simulink model "NewBlockFlow"  (R2021a)
settings: Solver=VariableStepAuto  StartTime=0.0  StopTime=10.0  RelTol=1e-3
values from neighbouring files (symbols this model uses):
  a = 0    [gainMaxDef.m]    (also in plot2.m = 2; simulink_test.m = 5)
  alpha = 1.195    [gainMaxDef.m]    (also in plot2.m = 1.9; simulink_test.m = 1.192)
  betac = 2    [plot2.m]    (also in simulink_test.m = 10)
  delay = 0.5    [plot2.m]    (also in simulink_test.m = 0.015)
  delay_a = 0.150    (= 0.15)    [plot2.m]    (also in simulink_test.m = 0.01)
  gnet = 40    [plot2.m]    (also in simulink_test.m = gnetset(k))
  omega = omegalist(l)    [gainMaxDef.m]    (also in plot2.m = 300; simulink_test.m = 0.8)
  omegader = 80    [simulink_test.m]
libraries: cstblocks x24, simulink x2
(part 1 of 2)
settings Model: Creator=shiva  LastModifiedBy=shiva

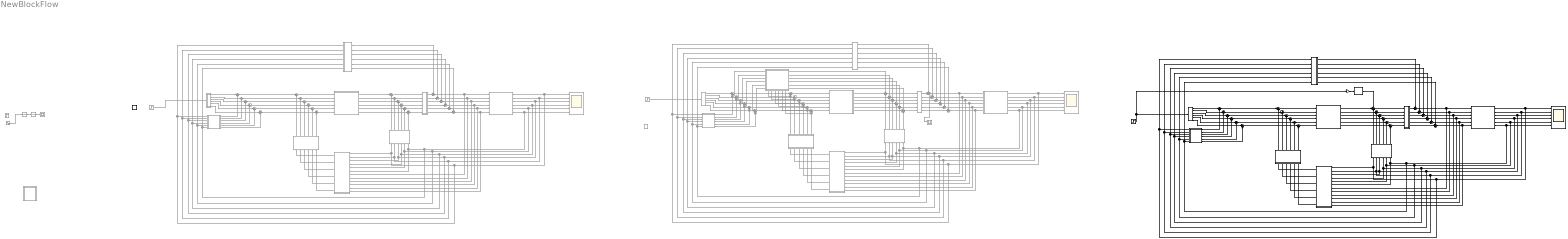
== system NewBlockFlow ==
  note: FLOW V3
  note: FLOW V2
  note: FLOW V1
  note: CONTROL BLOCK
  note: FEEDBACK
  note: INPUT AREA
  note: FEEDBACK
  note: CONTROL BLOCK
  note: INPUT AREA
  note: FEEDBACK
  note: CONTROL BLOCK
  note: INPUT AREA
  Adjency : Subsystem  Commented=on
  Adjency1 : Subsystem  Commented=on
  Adjency2 : Subsystem
  B : Subsystem  Commented=on
  B1 : Subsystem  Commented=on
  B2 : Subsystem
  C(s) : Subsystem  Commented=on
  C(s)1 : Subsystem  Commented=on
  C(s)2 : Subsystem
  CDOB_Subsys1 : Subsystem  Commented=on
  CDOB_Subsys2 : Subsystem
  CDOB_Subsys4 : Subsystem  Commented=on
  DSRdelayV2 : Subsystem
  Degree : Subsystem  Commented=on
  Degree1 : Subsystem  Commented=on
  Degree2 : Subsystem
  DerivativeEstimater : Subsystem  Commented=on
  DerivativeEstimater1 : Subsystem  Commented=on
  DerivativeEstimater2 : Subsystem
  G(s)e^(-tau*s) : Subsystem  Commented=on
  G(s)e^(-tau*s)1 : Subsystem  Commented=on
  G(s)e^(-tau*s)2 : Subsystem
  Gain : Gain  Gain=betac
  Identity : Subsystem  Commented=on
  PseudoDerivative : Subsystem  Commented=on
  Ramp : simulink/Sources/Ramp  slope=1  start=0  InitialOutput=0
  Ramp1 : simulink/Sources/Ramp  Commented=on  slope=1  start=0  InitialOutput=0
  Scope : Scope  Commented=on
  Scope1 : Scope  Commented=on  NumInputPorts=6
  Scope2 : Scope  Commented=on  NumInputPorts=2
  Scope3 : Scope  NumInputPorts=6
  Scope5 : Scope  Commented=on  NumInputPorts=6
  Sine Wave : Sin  Commented=on  SampleTime=0
  StateDerivative1 : Subsystem
  StateDerivative3 : Subsystem  Commented=on
  Step : Step  Commented=on  Time=0  SampleTime=0
  Step1 : Step  Commented=on  SampleTime=0
  Step2 : Step  Commented=on  Time=0  SampleTime=0
  Step3 : Step  Time=0  SampleTime=0
  Sum{,1..5,12..17,28..33} (18 alike) : Sum  Commented=on  Inputs=|++
  Sum{6..11,26..27,44..47} (12 alike) : Sum  Commented=on  Inputs=++|
  Sum{18..23,34..35,37..40} (12 alike) : Sum  Commented=on  Inputs=|-+
  Sum{24..25,36,41..43} (6 alike) : Sum  Commented=on  Inputs=-++
  Sum48 : Sum  Inputs=-++
  Sum{49,52..57,60,65..67} (11 alike) : Sum  Inputs=|++
  Sum{50..51,68..71} (6 alike) : Sum  Inputs=++|
  Sum{58..59,61..64} (6 alike) : Sum  Inputs=|-+
  beta*(DXc-Ax)*F(s) : Subsystem  Commented=on
      settings: PortSchema="{\"entries\":[{\"content\":{\"sides\":[{\"content\":{\"connectorIds\":[\"In1\",\"In2\",\"In3\",\"In4\",\"In5\",\"In6\"]},\"type\":\"ConnectorPlacement.EquallySpacedRectSide\",\"uuid\":\"7b965991-8f4b-4d23-8dac-1fc1cf204da0\"},{\"content\":{\"connectorIds\":[\"Out1\",\"Out2\",\"Out3\",\"Out4\",\"Out5\",\"Out6\"],\"side\":\"RIGHT\"},\"type\":\"ConnectorPlacement.EquallySpacedRectSide\",\"uuid\":\"f5ccf5a4-70bb-4fce-9767-13471ee96b32\"},{\"content\":{\"connectorIds\":[],\"side\":\"TOP\"},\"type\":\"ConnectorPlacement.EquallySpacedRectSide\",\"uuid\":\"af7cab47-c5e2-4c4a-b9c2-1fd2a05ea20b\"},{\"content\":{\"connectorIds\":[\"In7\",\"In8\",\"In9\",\"In10\",\"In11\",\"In12\"],\"side\":\"BOTTOM\"},\"type\":\"ConnectorPlacement.EquallySpacedRectSide\",\"uuid\":\"30ff81f8-6ce8-42b1-8056-7bce911790b7\"}]},\"type\":\"ConnectorPlacement.EquallySpacedConnector\",\"uuid\":\"9d803241-f085-403f-8915-bf1fb56b5898\"}],\"packageUris\":[\"http://schema.mathworks.com/mf0/Connector/R2020b\"],\"version\":\"1.0\"}"
  gain 1/a : Subsystem  Commented=on
  gain 1/a1 : Subsystem  Commented=on
  gain 1/a2 : Subsystem
  pseudoDer : TransferFcn  Commented=on  Numerator=[omegader 0]  Denominator=[1 omegader]
  pseudoDer1 : TransferFcn  Commented=on  Numerator=[omegader 0]  Denominator=[1 omegader]
  wires:
  G(s)e^(-tau*s)/1(pos) -> CDOB_Subsys4/1(XRes), DerivativeEstimater/1(pos), PseudoDerivative/1(Input), Adjency/1(Input), Scope5/1
  G(s)e^(-tau*s)/2(pos1) -> Scope5/2, PseudoDerivative/2(Input1), Adjency/2(Input1), CDOB_Subsys4/2(XRes1), DerivativeEstimater/2(pos1)
  G(s)e^(-tau*s)/3(pos2) -> Scope5/3, PseudoDerivative/3(Input2), Adjency/3(Input2), CDOB_Subsys4/3(XRes2), DerivativeEstimater/3(pos2)
  G(s)e^(-tau*s)/4(pos3) -> Scope5/4, PseudoDerivative/4(Input3), Adjency/4(Input3), CDOB_Subsys4/4(XRes3), DerivativeEstimater/4(pos3)
  G(s)e^(-tau*s)/5(pos4) -> Scope5/5, Adjency/5(Input4), PseudoDerivative/5(Input4), CDOB_Subsys4/5(XRes4), DerivativeEstimater/5(pos4)
  G(s)e^(-tau*s)/6(pos5) -> Scope5/6, CDOB_Subsys4/6(XRes5), DerivativeEstimater/6(pos5), PseudoDerivative/6(Input5), Adjency/6(Input5)
  DerivativeEstimater/1(est) -> Sum/2
  C(s)/1(Out1) -> Sum/1
  Sum6/1 -> CDOB_Subsys4/7(Acc.), G(s)e^(-tau*s)/1(In1)
  Sum7/1 -> CDOB_Subsys4/8(Acc.1), G(s)e^(-tau*s)/2(In2)
  C(s)/2(Out2) -> Sum1/1
  DerivativeEstimater/3(est2) -> Sum2/2
  C(s)/3(Out3) -> Sum2/1
  Sum8/1 -> CDOB_Subsys4/9(Acc.2), G(s)e^(-tau*s)/3(In3)
  DerivativeEstimater/4(est3) -> Sum3/2
  Sum9/1 -> CDOB_Subsys4/10(Acc.3), G(s)e^(-tau*s)/4(In4)
  C(s)/4(Out4) -> Sum3/1
  DerivativeEstimater/5(est4) -> Sum4/2
  C(s)/5(Out5) -> Sum4/1
  Sum10/1 -> CDOB_Subsys4/11(Acc.4), G(s)e^(-tau*s)/5(In5)
  DerivativeEstimater/6(est5) -> Sum5/2
  C(s)/6(Out6) -> Sum5/1
  Sum11/1 -> CDOB_Subsys4/12(Acc.5), G(s)e^(-tau*s)/6(In6)
  DerivativeEstimater/2(est1) -> Sum1/2
  gain 1/a/1(Out1) -> Sum6/2
  gain 1/a/2(Out2) -> Sum7/2
  gain 1/a/3(Out3) -> Sum8/2
  gain 1/a/4(Out4) -> Sum9/2
  gain 1/a/5(Out5) -> Sum10/2
  gain 1/a/6(Out6) -> Sum11/2
  Sum/1 -> gain 1/a/1(In1)
  Sum1/1 -> gain 1/a/2(In2)
  Sum2/1 -> gain 1/a/3(In3)
  Sum3/1 -> gain 1/a/4(In4)
  Sum4/1 -> gain 1/a/5(In5)
  Sum5/1 -> gain 1/a/6(In6)
  Step/1 -> B/1(Input)
  B/1(Output) -> Sum12/1
  Adjency/1(Output) -> Sum12/2
  B/2(Output1) -> Sum13/1
  B/3(Output2) -> Sum14/1
  B/4(Output3) -> Sum15/1
  B/5(Output4) -> Sum16/1
  B/6(Output5) -> Sum17/1
  Adjency/2(Output1) -> Sum13/2
  Adjency/3(Output2) -> Sum14/2
  Adjency/4(Output3) -> Sum15/2
  Adjency/5(Output4) -> Sum16/2
  Adjency/6(Output5) -> Sum17/2
  Sum12/1 -> Sum18/1
  Sum18/1 -> C(s)/1(R-F)
  Sum19/1 -> C(s)/2(R-F1)
  Sum20/1 -> C(s)/3(R-F2)
  Sum21/1 -> C(s)/4(R-F3)
  Sum22/1 -> C(s)/5(R-F4)
  Sum23/1 -> C(s)/6(R-F5)
  Sum13/1 -> Sum19/1
  Sum14/1 -> Sum20/1
  Sum15/1 -> Sum21/1
  Sum16/1 -> Sum22/1
  Sum17/1 -> Sum23/1
  CDOB_Subsys4/1(FeedBack) -> Degree/1(Input)
  CDOB_Subsys4/2(FeedBack1) -> Degree/2(Input1)
  CDOB_Subsys4/3(FeedBack2) -> Degree/3(Input2)
  CDOB_Subsys4/4(FeedBack3) -> Degree/4(Input3)
  CDOB_Subsys4/5(FeedBack4) -> Degree/5(Input4)
  CDOB_Subsys4/6(FeedBack5) -> Degree/6(Input5)
  Degree/1(Output) -> Sum18/2
  Degree/6(Output5) -> Sum23/2
  Degree/5(Output4) -> Sum22/2
  Degree/4(Output3) -> Sum21/2
  Degree/3(Output2) -> Sum20/2
  Degree/2(Output1) -> Sum19/2
  PseudoDerivative/1(Output) -> Sum6/1
  PseudoDerivative/2(Output1) -> Sum7/1
  PseudoDerivative/3(Output2) -> Sum8/1
  PseudoDerivative/4(Output3) -> Sum9/1
  PseudoDerivative/5(Output4) -> Sum10/1
  PseudoDerivative/6(Output5) -> Sum11/1
  pseudoDer/1 -> pseudoDer1/1
  pseudoDer1/1 -> Scope/1
  Sine Wave/1 -> pseudoDer/1
  Step2/1 -> B1/1(Input)
  StateDerivative3/1(Out1) -> Sum44/1
  StateDerivative3/6(Out6) -> Sum27/1
  StateDerivative3/3(Out3) -> Sum46/1
  StateDerivative3/2(Out2) -> Sum45/1
  Degree1/2(Output1) -> beta*(DXc-Ax)*F(s)/8(Input7), Sum35/2
  CDOB_Subsys1/6(FeedBack5) -> Degree1/6(Input5)
  Adjency1/5(Output4) -> beta*(DXc-Ax)*F(s)/5(Input4), Sum32/2
  B1/4(Output3) -> Sum31/1
  StateDerivative3/5(Out5) -> Sum26/1
  B1/1(Output) -> Sum28/1
  Sum34/1 -> C(s)1/1(R-F)
  Sum32/1 -> Sum39/1
  Degree1/5(Output4) -> beta*(DXc-Ax)*F(s)/11(Input10), Sum39/2
  Adjency1/3(Output2) -> beta*(DXc-Ax)*F(s)/3(Input2), Sum30/2
  B1/2(Output1) -> Sum29/1
  Sum38/1 -> C(s)1/4(R-F3)
  B1/6(Output5) -> Sum33/1
  Sum29/1 -> Sum35/1
  Adjency1/4(Output3) -> beta*(DXc-Ax)*F(s)/4(Input3), Sum31/2
  Sum30/1 -> Sum37/1
  Sum33/1 -> Sum40/1
  B1/5(Output4) -> Sum32/1
  Adjency1/2(Output1) -> beta*(DXc-Ax)*F(s)/2(Input1), Sum29/2
  Sum40/1 -> C(s)1/6(R-F5)
  G(s)e^(-tau*s)1/5(pos4) -> Scope1/5, Adjency1/5(Input4), StateDerivative3/5(Input4), CDOB_Subsys1/5(XRes4), DerivativeEstimater1/5(pos4)
  Sum27/1 -> CDOB_Subsys1/12(Acc.5), G(s)e^(-tau*s)1/6(In6)
  G(s)e^(-tau*s)1/3(pos2) -> Scope1/3, StateDerivative3/3(Input2), Adjency1/3(Input2), CDOB_Subsys1/3(XRes2), DerivativeEstimater1/3(pos2)
  Degree1/6(Output5) -> beta*(DXc-Ax)*F(s)/12(Input11), Sum40/2
  G(s)e^(-tau*s)1/4(pos3) -> Scope1/4, StateDerivative3/4(Input3), Adjency1/4(Input3), CDOB_Subsys1/4(XRes3), DerivativeEstimater1/4(pos3)
  G(s)e^(-tau*s)1/1(pos) -> CDOB_Subsys1/1(XRes), DerivativeEstimater1/1(pos), StateDerivative3/1(Input), Adjency1/1(Input), Scope1/1
  Sum47/1 -> CDOB_Subsys1/10(Acc.3), G(s)e^(-tau*s)1/4(In4)
  Degree1/4(Output3) -> beta*(DXc-Ax)*F(s)/10(Input9), Sum38/2
  CDOB_Subsys1/2(FeedBack1) -> Degree1/2(Input1)
  gain 1/a1/3(Out3) -> Sum46/2
  G(s)e^(-tau*s)1/6(pos5) -> Scope1/6, CDOB_Subsys1/6(XRes5), DerivativeEstimater1/6(pos5), StateDerivative3/6(Input5), Adjency1/6(Input5)
  gain 1/a1/6(Out6) -> Sum27/2
  Sum31/1 -> Sum38/1
  gain 1/a1/2(Out2) -> Sum45/2
  Sum28/1 -> Sum34/1
  Sum26/1 -> CDOB_Subsys1/11(Acc.4), G(s)e^(-tau*s)1/5(In5)
  Sum45/1 -> CDOB_Subsys1/8(Acc.1), G(s)e^(-tau*s)1/2(In2)
  Degree1/1(Output) -> beta*(DXc-Ax)*F(s)/7(Input6), Sum34/2
  Sum24/1 -> gain 1/a1/1(In1)
  Sum46/1 -> CDOB_Subsys1/9(Acc.2), G(s)e^(-tau*s)1/3(In3)
  StateDerivative3/4(Out4) -> Sum47/1
  CDOB_Subsys1/4(FeedBack3) -> Degree1/4(Input3)
  Sum39/1 -> C(s)1/5(R-F4)
  B1/3(Output2) -> Sum30/1
  Sum37/1 -> C(s)1/3(R-F2)
  G(s)e^(-tau*s)1/2(pos1) -> Scope1/2, StateDerivative3/2(Input1), Adjency1/2(Input1), CDOB_Subsys1/2(XRes1), DerivativeEstimater1/2(pos1)
  gain 1/a1/1(Out1) -> Sum44/2
  CDOB_Subsys1/3(FeedBack2) -> Degree1/3(Input2)
  Degree1/3(Output2) -> beta*(DXc-Ax)*F(s)/9(Input8), Sum37/2
  gain 1/a1/4(Out4) -> Sum47/2
  Sum44/1 -> Scope2/1, CDOB_Subsys1/7(Acc.), G(s)e^(-tau*s)1/1(In1)
  Sum35/1 -> C(s)1/2(R-F1)
  CDOB_Subsys1/1(FeedBack) -> Degree1/1(Input)
  gain 1/a1/5(Out5) -> Sum26/2
  CDOB_Subsys1/5(FeedBack4) -> Degree1/5(Input4)
  Adjency1/1(Output) -> beta*(DXc-Ax)*F(s)/1(Input), Sum28/2
  Adjency1/6(Output5) -> beta*(DXc-Ax)*F(s)/6(Input5), Sum33/2
  Sum43/1 -> gain 1/a1/6(In6)
  Sum25/1 -> gain 1/a1/2(In2)
  Sum36/1 -> gain 1/a1/3(In3)
  Sum41/1 -> gain 1/a1/4(In4)
  Sum42/1 -> gain 1/a1/5(In5)
  beta*(DXc-Ax)*F(s)/1(Output) -> Sum24/1
  DerivativeEstimater1/1(est) -> Sum24/3
  DerivativeEstimater1/6(est5) -> Sum43/3
  C(s)1/6(Out6) -> Sum43/2
  DerivativeEstimater1/5(est4) -> Sum42/3
  C(s)1/5(Out5) -> Sum42/2
  C(s)1/4(Out4) -> Sum41/2
  DerivativeEstimater1/4(est3) -> Sum41/3
  DerivativeEstimater1/3(est2) -> Sum36/3
  C(s)1/3(Out3) -> Sum36/2
  DerivativeEstimater1/2(est1) -> Sum25/3
  C(s)1/2(Out2) -> Sum25/2
  C(s)1/1(Out1) -> Sum24/2
  beta*(DXc-Ax)*F(s)/2(Output1) -> Sum25/1
  beta*(DXc-Ax)*F(s)/3(Output2) -> Sum36/1
  beta*(DXc-Ax)*F(s)/4(Output3) -> Sum41/1
  beta*(DXc-Ax)*F(s)/5(Output4) -> Sum42/1
  beta*(DXc-Ax)*F(s)/6(Output5) -> Sum43/1
  Step3/1 -> Gain/1, B2/1(Input)
  StateDerivative1/1(Out1) -> Sum68/1
  StateDerivative1/6(Out6) -> Sum51/1
  StateDerivative1/3(Out3) -> Sum70/1
  StateDerivative1/2(Out2) -> Sum69/1
  Degree2/2(Output1) -> Sum59/2
  CDOB_Subsys2/6(FeedBack5) -> Degree2/6(Input5)
  Adjency2/5(Output4) -> Sum56/2
  B2/4(Output3) -> Sum55/1
  StateDerivative1/5(Out5) -> Sum50/1
  B2/1(Output) -> Sum52/1
  Sum58/1 -> C(s)2/1(R-F)
  Sum56/1 -> Sum63/1
  Degree2/5(Output4) -> Sum63/2
  Adjency2/3(Output2) -> Sum54/2
  B2/2(Output1) -> Sum53/1
  Sum62/1 -> C(s)2/4(R-F3)
  B2/6(Output5) -> Sum57/1
  Sum53/1 -> Sum59/1
  Adjency2/4(Output3) -> Sum55/2
  Sum54/1 -> Sum61/1
  Sum57/1 -> Sum64/1
  B2/5(Output4) -> Sum56/1
  Adjency2/2(Output1) -> Sum53/2
  Sum64/1 -> C(s)2/6(R-F5)
  Sum66/1 -> gain 1/a2/5(In5)
  G(s)e^(-tau*s)2/5(pos4) -> Scope3/5, Adjency2/5(Input4), StateDerivative1/5(Input4), CDOB_Subsys2/5(XRes4), DerivativeEstimater2/5(pos4)
  DerivativeEstimater2/6(est5) -> Sum67/2
  C(s)2/5(Out5) -> Sum66/1
  Sum51/1 -> CDOB_Subsys2/12(Acc.5), G(s)e^(-tau*s)2/6(In6)
  G(s)e^(-tau*s)2/3(pos2) -> Scope3/3, StateDerivative1/3(Input2), Adjency2/3(Input2), CDOB_Subsys2/3(XRes2), DerivativeEstimater2/3(pos2)
  C(s)2/2(Out2) -> Sum49/1
  Degree2/6(Output5) -> Sum64/2
  G(s)e^(-tau*s)2/4(pos3) -> Scope3/4, StateDerivative1/4(Input3), Adjency2/4(Input3), CDOB_Subsys2/4(XRes3), DerivativeEstimater2/4(pos3)
  G(s)e^(-tau*s)2/1(pos) -> CDOB_Subsys2/1(XRes), DerivativeEstimater2/1(pos), StateDerivative1/1(Input), Adjency2/1(Input), Scope3/1
  DerivativeEstimater2/2(est1) -> Sum49/2
  Sum71/1 -> CDOB_Subsys2/10(Acc.3), G(s)e^(-tau*s)2/4(In4)
  Sum60/1 -> gain 1/a2/3(In3)
  Degree2/4(Output3) -> Sum62/2
  DerivativeEstimater2/3(est2) -> Sum60/2
  Sum49/1 -> gain 1/a2/2(In2)
  CDOB_Subsys2/2(FeedBack1) -> Degree2/2(Input1)
  C(s)2/3(Out3) -> Sum60/1
  gain 1/a2/3(Out3) -> Sum70/2
  G(s)e^(-tau*s)2/6(pos5) -> Scope3/6, CDOB_Subsys2/6(XRes5), DerivativeEstimater2/6(pos5), StateDerivative1/6(Input5), Adjency2/6(Input5)
  Sum65/1 -> gain 1/a2/4(In4)
  gain 1/a2/6(Out6) -> Sum51/2
  C(s)2/4(Out4) -> Sum65/1
  Sum55/1 -> Sum62/1
  gain 1/a2/2(Out2) -> Sum69/2
  Sum52/1 -> Sum58/1
  Sum50/1 -> CDOB_Subsys2/11(Acc.4), G(s)e^(-tau*s)2/5(In5)
  Sum69/1 -> CDOB_Subsys2/8(Acc.1), G(s)e^(-tau*s)2/2(In2)
  Degree2/1(Output) -> Sum58/2
  Sum67/1 -> gain 1/a2/6(In6)
  Sum48/1 -> gain 1/a2/1(In1)
  Sum70/1 -> CDOB_Subsys2/9(Acc.2), G(s)e^(-tau*s)2/3(In3)
  StateDerivative1/4(Out4) -> Sum71/1
  CDOB_Subsys2/4(FeedBack3) -> Degree2/4(Input3)
  Sum63/1 -> C(s)2/5(R-F4)
  B2/3(Output2) -> Sum54/1
  DerivativeEstimater2/4(est3) -> Sum65/2
  Sum61/1 -> C(s)2/3(R-F2)
  G(s)e^(-tau*s)2/2(pos1) -> Scope3/2, StateDerivative1/2(Input1), Adjency2/2(Input1), CDOB_Subsys2/2(XRes1), DerivativeEstimater2/2(pos1)
  gain 1/a2/1(Out1) -> Sum68/2
  CDOB_Subsys2/3(FeedBack2) -> Degree2/3(Input2)
  Degree2/3(Output2) -> Sum61/2
  gain 1/a2/4(Out4) -> Sum71/2
  Sum68/1 -> CDOB_Subsys2/7(Acc.), G(s)e^(-tau*s)2/1(In1)
  Sum59/1 -> C(s)2/2(R-F1)
  C(s)2/6(Out6) -> Sum67/1
  DerivativeEstimater2/5(est4) -> Sum66/2
  CDOB_Subsys2/1(FeedBack) -> Degree2/1(Input)
  gain 1/a2/5(Out5) -> Sum50/2
  CDOB_Subsys2/5(FeedBack4) -> Degree2/5(Input4)
  Adjency2/1(Output) -> Sum52/2
  Adjency2/6(Output5) -> Sum57/2
  Gain/1 -> DSRdelayV2/1(Input)
  C(s)2/1(Out1) -> Sum48/2
  DerivativeEstimater2/1(est) -> Sum48/3
  DSRdelayV2/1(est) -> Sum48/1

== system NewBlockFlow/Adjency ==
  Input : Inport
  Input1 : Inport  Port=2
  Input2 : Inport  Port=3
  Input3 : Inport  Port=4
  Input4 : Inport  Port=5
  Input5 : Inport  Port=6
  Sum : Sum  Inputs=|++
  Sum1 : Sum  Inputs=|++
  Sum2 : Sum  Inputs=++++
  Terminator : Terminator
  Zero : Constant  Value=0  OutDataTypeStr=Inherit: Inherit via back propagation
  Output : Outport
  Output1 : Outport  Port=2
  Output2 : Outport  Port=3
  Output3 : Outport  Port=4
  Output4 : Outport  Port=5
  Output5 : Outport  Port=6
  wires:
  Input2/1 -> Sum2/2, Output4/1, Sum/2
  Input1/1 -> Sum2/1, Output3/1, Sum1/2
  Sum/1 -> Output1/1
  Input3/1 -> Sum2/3
  Input4/1 -> Sum2/4
  Input/1 -> Sum/1, Sum1/1
  Sum1/1 -> Output2/1
  Zero/1 -> Output/1
  Input5/1 -> Terminator/1
  Sum2/1 -> Output5/1

== system NewBlockFlow/Adjency1 ==
  Input : Inport
  Input1 : Inport  Port=2
  Input2 : Inport  Port=3
  Input3 : Inport  Port=4
  Input4 : Inport  Port=5
  Input5 : Inport  Port=6
  Sum : Sum  Inputs=|++
  Sum1 : Sum  Inputs=|++
  Sum2 : Sum  Inputs=++++
  Terminator : Terminator
  Zero : Constant  Value=0  OutDataTypeStr=Inherit: Inherit via back propagation
  Output : Outport
  Output1 : Outport  Port=2
  Output2 : Outport  Port=3
  Output3 : Outport  Port=4
  Output4 : Outport  Port=5
  Output5 : Outport  Port=6
  wires:
  Input2/1 -> Sum2/2, Output4/1, Sum/2
  Input1/1 -> Sum2/1, Output3/1, Sum1/2
  Sum/1 -> Output1/1
  Input3/1 -> Sum2/3
  Input4/1 -> Sum2/4
  Input/1 -> Sum/1, Sum1/1
  Sum1/1 -> Output2/1
  Zero/1 -> Output/1
  Input5/1 -> Terminator/1
  Sum2/1 -> Output5/1

== system NewBlockFlow/Adjency2 ==
  Input : Inport
  Input1 : Inport  Port=2
  Input2 : Inport  Port=3
  Input3 : Inport  Port=4
  Input4 : Inport  Port=5
  Input5 : Inport  Port=6
  Sum : Sum  Inputs=|++
  Sum1 : Sum  Inputs=|++
  Sum2 : Sum  Inputs=++++
  Terminator : Terminator
  Zero : Constant  Value=0  OutDataTypeStr=Inherit: Inherit via back propagation
  Output : Outport
  Output1 : Outport  Port=2
  Output2 : Outport  Port=3
  Output3 : Outport  Port=4
  Output4 : Outport  Port=5
  Output5 : Outport  Port=6
  wires:
  Input2/1 -> Sum2/2, Output4/1, Sum/2
  Input1/1 -> Sum2/1, Output3/1, Sum1/2
  Sum/1 -> Output1/1
  Input3/1 -> Sum2/3
  Input4/1 -> Sum2/4
  Input/1 -> Sum/1, Sum1/1
  Sum1/1 -> Output2/1
  Zero/1 -> Output/1
  Input5/1 -> Terminator/1
  Sum2/1 -> Output5/1

== system NewBlockFlow/B ==
  Input : Inport
  Zero : Constant  Value=0  OutDataTypeStr=Inherit: Inherit via back propagation
  Output : Outport
  Output1 : Outport  Port=2
  Output2 : Outport  Port=3
  Output3 : Outport  Port=4
  Output4 : Outport  Port=5
  Output5 : Outport  Port=6
  wires:
  Zero/1 -> Output5/1, Output4/1, Output3/1, Output2/1, Output1/1
  Input/1 -> Output/1

== system NewBlockFlow/B1 ==
  Input : Inport
  Zero : Constant  Value=0  OutDataTypeStr=Inherit: Inherit via back propagation
  Output : Outport
  Output1 : Outport  Port=2
  Output2 : Outport  Port=3
  Output3 : Outport  Port=4
  Output4 : Outport  Port=5
  Output5 : Outport  Port=6
  wires:
  Zero/1 -> Output5/1, Output4/1, Output3/1, Output2/1, Output1/1
  Input/1 -> Output/1

== system NewBlockFlow/B2 ==
  Input : Inport
  Zero : Constant  Value=0  OutDataTypeStr=Inherit: Inherit via back propagation
  Output : Outport
  Output1 : Outport  Port=2
  Output2 : Outport  Port=3
  Output3 : Outport  Port=4
  Output4 : Outport  Port=5
  Output5 : Outport  Port=6
  wires:
  Zero/1 -> Output5/1, Output4/1, Output3/1, Output2/1, Output1/1
  Input/1 -> Output/1

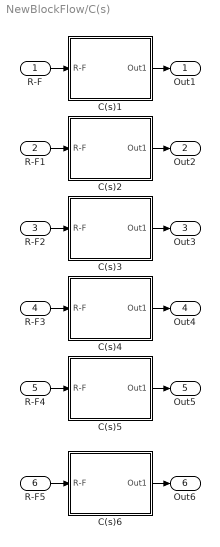
== system NewBlockFlow/C(s) ==
  R-F : Inport
  R-F1 : Inport  Port=2
  R-F2 : Inport  Port=3
  R-F3 : Inport  Port=4
  R-F4 : Inport  Port=5
  R-F5 : Inport  Port=6
  C(s)1 : Subsystem
  C(s)2 : Subsystem
  C(s)3 : Subsystem
  C(s)4 : Subsystem
  C(s)5 : Subsystem
  C(s)6 : Subsystem
  Out1 : Outport
  Out2 : Outport  Port=2
  Out3 : Outport  Port=3
  Out4 : Outport  Port=4
  Out5 : Outport  Port=5
  Out6 : Outport  Port=6
  wires:
  R-F4/1 -> C(s)5/1(R-F)
  R-F2/1 -> C(s)3/1(R-F)
  C(s)3/1(Out1) -> Out3/1
  R-F1/1 -> C(s)2/1(R-F)
  C(s)4/1(Out1) -> Out4/1
  C(s)6/1(Out1) -> Out6/1
  R-F3/1 -> C(s)4/1(R-F)
  C(s)1/1(Out1) -> Out1/1
  R-F5/1 -> C(s)6/1(R-F)
  R-F/1 -> C(s)1/1(R-F)
  C(s)2/1(Out1) -> Out2/1
  C(s)5/1(Out1) -> Out5/1

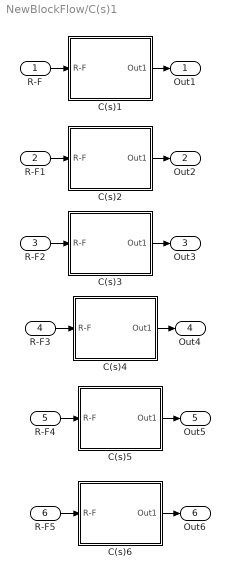
== system NewBlockFlow/C(s)1 ==
  R-F : Inport
  R-F1 : Inport  Port=2
  R-F2 : Inport  Port=3
  R-F3 : Inport  Port=4
  R-F4 : Inport  Port=5
  R-F5 : Inport  Port=6
  C(s)1 : Subsystem
  C(s)2 : Subsystem
  C(s)3 : Subsystem
  C(s)4 : Subsystem
  C(s)5 : Subsystem
  C(s)6 : Subsystem
  Out1 : Outport
  Out2 : Outport  Port=2
  Out3 : Outport  Port=3
  Out4 : Outport  Port=4
  Out5 : Outport  Port=5
  Out6 : Outport  Port=6
  wires:
  C(s)1/1(Out1) -> Out1/1
  R-F/1 -> C(s)1/1(R-F)
  C(s)2/1(Out1) -> Out2/1
  R-F1/1 -> C(s)2/1(R-F)
  C(s)3/1(Out1) -> Out3/1
  R-F2/1 -> C(s)3/1(R-F)
  C(s)4/1(Out1) -> Out4/1
  R-F3/1 -> C(s)4/1(R-F)
  C(s)5/1(Out1) -> Out5/1
  R-F4/1 -> C(s)5/1(R-F)
  C(s)6/1(Out1) -> Out6/1
  R-F5/1 -> C(s)6/1(R-F)

== system NewBlockFlow/C(s)2 ==
  R-F : Inport
  R-F1 : Inport  Port=2
  R-F2 : Inport  Port=3
  R-F3 : Inport  Port=4
  R-F4 : Inport  Port=5
  R-F5 : Inport  Port=6
  C(s)1 : Subsystem
  C(s)2 : Subsystem
  C(s)3 : Subsystem
  C(s)4 : Subsystem
  C(s)5 : Subsystem
  C(s)6 : Subsystem
  Out1 : Outport
  Out2 : Outport  Port=2
  Out3 : Outport  Port=3
  Out4 : Outport  Port=4
  Out5 : Outport  Port=5
  Out6 : Outport  Port=6
  wires:
  C(s)1/1(Out1) -> Out1/1
  R-F/1 -> C(s)1/1(R-F)
  C(s)2/1(Out1) -> Out2/1
  R-F1/1 -> C(s)2/1(R-F)
  C(s)3/1(Out1) -> Out3/1
  R-F2/1 -> C(s)3/1(R-F)
  C(s)4/1(Out1) -> Out4/1
  R-F3/1 -> C(s)4/1(R-F)
  C(s)5/1(Out1) -> Out5/1
  R-F4/1 -> C(s)5/1(R-F)
  C(s)6/1(Out1) -> Out6/1
  R-F5/1 -> C(s)6/1(R-F)

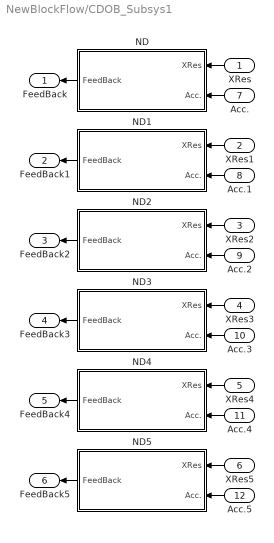
== system NewBlockFlow/CDOB_Subsys1 ==
  XRes : Inport
  XRes1 : Inport  Port=2
  XRes2 : Inport  Port=3
  XRes3 : Inport  Port=4
  XRes4 : Inport  Port=5
  XRes5 : Inport  Port=6
  Acc. : Inport  Port=7
  Acc.1 : Inport  Port=8
  Acc.2 : Inport  Port=9
  Acc.3 : Inport  Port=10
  Acc.4 : Inport  Port=11
  Acc.5 : Inport  Port=12
  ND : Subsystem
  ND1 : Subsystem
  ND2 : Subsystem
  ND3 : Subsystem
  ND4 : Subsystem
  ND5 : Subsystem
  FeedBack : Outport
  FeedBack1 : Outport  Port=2
  FeedBack2 : Outport  Port=3
  FeedBack3 : Outport  Port=4
  FeedBack4 : Outport  Port=5
  FeedBack5 : Outport  Port=6
  wires:
  Acc./1 -> ND/2(Acc.)
  XRes/1 -> ND/1(XRes)
  Acc.4/1 -> ND4/2(Acc.)
  Acc.3/1 -> ND3/2(Acc.)
  XRes1/1 -> ND1/1(XRes)
  XRes2/1 -> ND2/1(XRes)
  XRes4/1 -> ND4/1(XRes)
  XRes5/1 -> ND5/1(XRes)
  Acc.2/1 -> ND2/2(Acc.)
  ND5/1(FeedBack) -> FeedBack5/1
  ND1/1(FeedBack) -> FeedBack1/1
  ND2/1(FeedBack) -> FeedBack2/1
  Acc.5/1 -> ND5/2(Acc.)
  ND4/1(FeedBack) -> FeedBack4/1
  ND/1(FeedBack) -> FeedBack/1
  ND3/1(FeedBack) -> FeedBack3/1
  XRes3/1 -> ND3/1(XRes)
  Acc.1/1 -> ND1/2(Acc.)

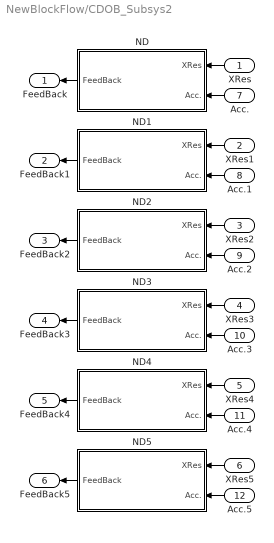
== system NewBlockFlow/CDOB_Subsys2 ==
  XRes : Inport
  XRes1 : Inport  Port=2
  XRes2 : Inport  Port=3
  XRes3 : Inport  Port=4
  XRes4 : Inport  Port=5
  XRes5 : Inport  Port=6
  Acc. : Inport  Port=7
  Acc.1 : Inport  Port=8
  Acc.2 : Inport  Port=9
  Acc.3 : Inport  Port=10
  Acc.4 : Inport  Port=11
  Acc.5 : Inport  Port=12
  ND : Subsystem
  ND1 : Subsystem
  ND2 : Subsystem
  ND3 : Subsystem
  ND4 : Subsystem
  ND5 : Subsystem
  FeedBack : Outport
  FeedBack1 : Outport  Port=2
  FeedBack2 : Outport  Port=3
  FeedBack3 : Outport  Port=4
  FeedBack4 : Outport  Port=5
  FeedBack5 : Outport  Port=6
  wires:
  Acc./1 -> ND/2(Acc.)
  XRes/1 -> ND/1(XRes)
  Acc.4/1 -> ND4/2(Acc.)
  Acc.3/1 -> ND3/2(Acc.)
  XRes1/1 -> ND1/1(XRes)
  XRes2/1 -> ND2/1(XRes)
  XRes4/1 -> ND4/1(XRes)
  XRes5/1 -> ND5/1(XRes)
  Acc.2/1 -> ND2/2(Acc.)
  ND5/1(FeedBack) -> FeedBack5/1
  ND1/1(FeedBack) -> FeedBack1/1
  ND2/1(FeedBack) -> FeedBack2/1
  Acc.5/1 -> ND5/2(Acc.)
  ND4/1(FeedBack) -> FeedBack4/1
  ND/1(FeedBack) -> FeedBack/1
  ND3/1(FeedBack) -> FeedBack3/1
  XRes3/1 -> ND3/1(XRes)
  Acc.1/1 -> ND1/2(Acc.)

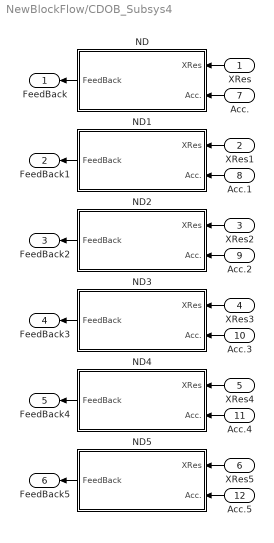
== system NewBlockFlow/CDOB_Subsys4 ==
  XRes : Inport
  XRes1 : Inport  Port=2
  XRes2 : Inport  Port=3
  XRes3 : Inport  Port=4
  XRes4 : Inport  Port=5
  XRes5 : Inport  Port=6
  Acc. : Inport  Port=7
  Acc.1 : Inport  Port=8
  Acc.2 : Inport  Port=9
  Acc.3 : Inport  Port=10
  Acc.4 : Inport  Port=11
  Acc.5 : Inport  Port=12
  ND : Subsystem
  ND1 : Subsystem
  ND2 : Subsystem
  ND3 : Subsystem
  ND4 : Subsystem
  ND5 : Subsystem
  FeedBack : Outport
  FeedBack1 : Outport  Port=2
  FeedBack2 : Outport  Port=3
  FeedBack3 : Outport  Port=4
  FeedBack4 : Outport  Port=5
  FeedBack5 : Outport  Port=6
  wires:
  Acc./1 -> ND/2(Acc.)
  XRes/1 -> ND/1(XRes)
  Acc.4/1 -> ND4/2(Acc.)
  Acc.3/1 -> ND3/2(Acc.)
  XRes1/1 -> ND1/1(XRes)
  XRes2/1 -> ND2/1(XRes)
  XRes4/1 -> ND4/1(XRes)
  XRes5/1 -> ND5/1(XRes)
  Acc.2/1 -> ND2/2(Acc.)
  ND5/1(FeedBack) -> FeedBack5/1
  ND1/1(FeedBack) -> FeedBack1/1
  ND2/1(FeedBack) -> FeedBack2/1
  Acc.5/1 -> ND5/2(Acc.)
  ND4/1(FeedBack) -> FeedBack4/1
  ND/1(FeedBack) -> FeedBack/1
  ND3/1(FeedBack) -> FeedBack3/1
  XRes3/1 -> ND3/1(XRes)
  Acc.1/1 -> ND1/2(Acc.)

== system NewBlockFlow/DSRdelayV2 ==
  Input : Inport
  Gain : Gain  Gain=1/delay
  Gain1 : Gain  Gain=1/delay
  Sum : Sum  Inputs=-+|
  Sum13 : Sum  Inputs=-+|
  Transfer Fcn : TransferFcn  Numerator=[omega]  Denominator=[1 omega]
  Transfer Fcn1 : TransferFcn  Numerator=[omega]  Denominator=[1 omega]
  Transport Delay : TransportDelay  DelayTime=delay
  Transport Delay13 : TransportDelay  DelayTime=delay
  est : Outport
  wires:
  Sum/1 -> Gain/1
  Gain/1 -> Transfer Fcn/1
  Transfer Fcn/1 -> Transport Delay13/1, Sum13/2
  Input/1 -> Transport Delay/1, Sum/2
  Transport Delay/1 -> Sum/1
  Transfer Fcn1/1 -> est/1
  Transport Delay13/1 -> Sum13/1
  Gain1/1 -> Transfer Fcn1/1
  Sum13/1 -> Gain1/1

== system NewBlockFlow/Degree ==
  Input : Inport
  Input1 : Inport  Port=2
  Input2 : Inport  Port=3
  Input3 : Inport  Port=4
  Input4 : Inport  Port=5
  Input5 : Inport  Port=6
  Gain : Gain  Gain=2
  Gain1 : Gain  Gain=2
  Gain4 : Gain  Gain=4
  Output : Outport
  Output1 : Outport  Port=2
  Output2 : Outport  Port=3
  Output3 : Outport  Port=4
  Output4 : Outport  Port=5
  Output5 : Outport  Port=6
  wires:
  Input3/1 -> Output3/1
  Input1/1 -> Gain/1
  Gain1/1 -> Output2/1
  Input2/1 -> Gain1/1
  Input/1 -> Output/1
  Input5/1 -> Gain4/1
  Gain4/1 -> Output5/1
  Gain/1 -> Output1/1
  Input4/1 -> Output4/1

== system NewBlockFlow/Degree1 ==
  Input : Inport
  Input1 : Inport  Port=2
  Input2 : Inport  Port=3
  Input3 : Inport  Port=4
  Input4 : Inport  Port=5
  Input5 : Inport  Port=6
  Gain : Gain  Gain=2
  Gain1 : Gain  Gain=2
  Gain4 : Gain  Gain=4
  Output : Outport
  Output1 : Outport  Port=2
  Output2 : Outport  Port=3
  Output3 : Outport  Port=4
  Output4 : Outport  Port=5
  Output5 : Outport  Port=6
  wires:
  Input3/1 -> Output3/1
  Input1/1 -> Gain/1
  Gain1/1 -> Output2/1
  Input2/1 -> Gain1/1
  Input/1 -> Output/1
  Input5/1 -> Gain4/1
  Gain4/1 -> Output5/1
  Gain/1 -> Output1/1
  Input4/1 -> Output4/1

== system NewBlockFlow/Degree2 ==
  Input : Inport
  Input1 : Inport  Port=2
  Input2 : Inport  Port=3
  Input3 : Inport  Port=4
  Input4 : Inport  Port=5
  Input5 : Inport  Port=6
  Gain : Gain  Gain=2
  Gain1 : Gain  Gain=2
  Gain4 : Gain  Gain=4
  Output : Outport
  Output1 : Outport  Port=2
  Output2 : Outport  Port=3
  Output3 : Outport  Port=4
  Output4 : Outport  Port=5
  Output5 : Outport  Port=6
  wires:
  Input3/1 -> Output3/1
  Input1/1 -> Gain/1
  Gain1/1 -> Output2/1
  Input2/1 -> Gain1/1
  Input/1 -> Output/1
  Input5/1 -> Gain4/1
  Gain4/1 -> Output5/1
  Gain/1 -> Output1/1
  Input4/1 -> Output4/1

== system NewBlockFlow/DerivativeEstimater ==
  pos : Inport
  pos1 : Inport  Port=2
  pos2 : Inport  Port=3
  pos3 : Inport  Port=4
  pos4 : Inport  Port=5
  pos5 : Inport  Port=6
  DSRdelayV1 : Subsystem
  DSRdelayV2 : Subsystem
  DSRdelayV3 : Subsystem
  DSRdelayV4 : Subsystem
  DSRdelayV5 : Subsystem
  DSRdelayV6 : Subsystem
  est : Outport
  est1 : Outport  Port=2
  est2 : Outport  Port=3
  est3 : Outport  Port=4
  est4 : Outport  Port=5
  est5 : Outport  Port=6
  wires:
  pos1/1 -> DSRdelayV1/1(Input)
  pos/1 -> DSRdelayV2/1(Input)
  DSRdelayV2/1(est) -> est/1
  pos2/1 -> DSRdelayV3/1(Input)
  pos3/1 -> DSRdelayV4/1(Input)
  pos4/1 -> DSRdelayV5/1(Input)
  pos5/1 -> DSRdelayV6/1(Input)
  DSRdelayV5/1(est) -> est4/1
  DSRdelayV6/1(est) -> est5/1
  DSRdelayV4/1(est) -> est3/1
  DSRdelayV3/1(est) -> est2/1
  DSRdelayV1/1(est) -> est1/1

== system NewBlockFlow/DerivativeEstimater1 ==
  pos : Inport
  pos1 : Inport  Port=2
  pos2 : Inport  Port=3
  pos3 : Inport  Port=4
  pos4 : Inport  Port=5
  pos5 : Inport  Port=6
  DSRdelayV1 : Subsystem
  DSRdelayV2 : Subsystem
  DSRdelayV3 : Subsystem
  DSRdelayV4 : Subsystem
  DSRdelayV5 : Subsystem
  DSRdelayV6 : Subsystem
  est : Outport
  est1 : Outport  Port=2
  est2 : Outport  Port=3
  est3 : Outport  Port=4
  est4 : Outport  Port=5
  est5 : Outport  Port=6
  wires:
  pos1/1 -> DSRdelayV1/1(Input)
  pos/1 -> DSRdelayV2/1(Input)
  DSRdelayV2/1(est) -> est/1
  pos2/1 -> DSRdelayV3/1(Input)
  pos3/1 -> DSRdelayV4/1(Input)
  pos4/1 -> DSRdelayV5/1(Input)
  pos5/1 -> DSRdelayV6/1(Input)
  DSRdelayV5/1(est) -> est4/1
  DSRdelayV6/1(est) -> est5/1
  DSRdelayV4/1(est) -> est3/1
  DSRdelayV3/1(est) -> est2/1
  DSRdelayV1/1(est) -> est1/1

== system NewBlockFlow/DerivativeEstimater2 ==
  pos : Inport
  pos1 : Inport  Port=2
  pos2 : Inport  Port=3
  pos3 : Inport  Port=4
  pos4 : Inport  Port=5
  pos5 : Inport  Port=6
  DSRdelayV1 : Subsystem
  DSRdelayV2 : Subsystem
  DSRdelayV3 : Subsystem
  DSRdelayV4 : Subsystem
  DSRdelayV5 : Subsystem
  DSRdelayV6 : Subsystem
  est : Outport
  est1 : Outport  Port=2
  est2 : Outport  Port=3
  est3 : Outport  Port=4
  est4 : Outport  Port=5
  est5 : Outport  Port=6
  wires:
  pos1/1 -> DSRdelayV1/1(Input)
  pos/1 -> DSRdelayV2/1(Input)
  DSRdelayV2/1(est) -> est/1
  pos2/1 -> DSRdelayV3/1(Input)
  pos3/1 -> DSRdelayV4/1(Input)
  pos4/1 -> DSRdelayV5/1(Input)
  pos5/1 -> DSRdelayV6/1(Input)
  DSRdelayV5/1(est) -> est4/1
  DSRdelayV6/1(est) -> est5/1
  DSRdelayV4/1(est) -> est3/1
  DSRdelayV3/1(est) -> est2/1
  DSRdelayV1/1(est) -> est1/1

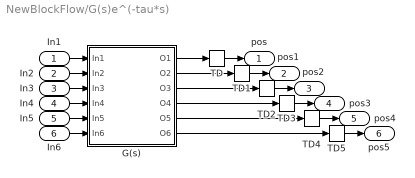
== system NewBlockFlow/G(s)e^(-tau*s) ==
  In1 : Inport
  In2 : Inport  Port=2
  In3 : Inport  Port=3
  In4 : Inport  Port=4
  In5 : Inport  Port=5
  In6 : Inport  Port=6
  G(s) : Subsystem
  TD{,1..5} (6 alike) : TransportDelay  DelayTime=delay_a
  pos : Outport
  pos1 : Outport  Port=2
  pos2 : Outport  Port=3
  pos3 : Outport  Port=4
  pos4 : Outport  Port=5
  pos5 : Outport  Port=6
  wires:
  G(s)/3(O3) -> TD2/1
  In4/1 -> G(s)/4(In4)
  G(s)/1(O1) -> TD/1
  TD4/1 -> pos4/1
  G(s)/4(O4) -> TD3/1
  G(s)/5(O5) -> TD4/1
  TD3/1 -> pos3/1
  G(s)/6(O6) -> TD5/1
  G(s)/2(O2) -> TD1/1
  In6/1 -> G(s)/6(In6)
  In2/1 -> G(s)/2(In2)
  In1/1 -> G(s)/1(In1)
  In3/1 -> G(s)/3(In3)
  TD2/1 -> pos2/1
  TD5/1 -> pos5/1
  TD1/1 -> pos1/1
  TD/1 -> pos/1
  In5/1 -> G(s)/5(In5)

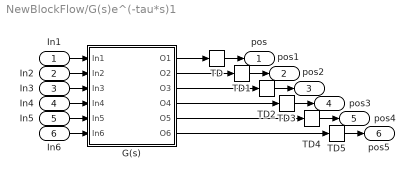
== system NewBlockFlow/G(s)e^(-tau*s)1 ==
  In1 : Inport
  In2 : Inport  Port=2
  In3 : Inport  Port=3
  In4 : Inport  Port=4
  In5 : Inport  Port=5
  In6 : Inport  Port=6
  G(s) : Subsystem
  TD{,1..5} (6 alike) : TransportDelay  DelayTime=delay_a
  pos : Outport
  pos1 : Outport  Port=2
  pos2 : Outport  Port=3
  pos3 : Outport  Port=4
  pos4 : Outport  Port=5
  pos5 : Outport  Port=6
  wires:
  G(s)/3(O3) -> TD2/1
  In4/1 -> G(s)/4(In4)
  G(s)/1(O1) -> TD/1
  TD4/1 -> pos4/1
  G(s)/4(O4) -> TD3/1
  G(s)/5(O5) -> TD4/1
  TD3/1 -> pos3/1
  G(s)/6(O6) -> TD5/1
  G(s)/2(O2) -> TD1/1
  In6/1 -> G(s)/6(In6)
  In2/1 -> G(s)/2(In2)
  In1/1 -> G(s)/1(In1)
  In3/1 -> G(s)/3(In3)
  TD2/1 -> pos2/1
  TD5/1 -> pos5/1
  TD1/1 -> pos1/1
  TD/1 -> pos/1
  In5/1 -> G(s)/5(In5)

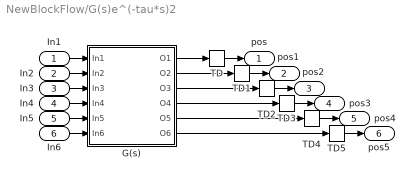
== system NewBlockFlow/G(s)e^(-tau*s)2 ==
  In1 : Inport
  In2 : Inport  Port=2
  In3 : Inport  Port=3
  In4 : Inport  Port=4
  In5 : Inport  Port=5
  In6 : Inport  Port=6
  G(s) : Subsystem
  TD{,1..5} (6 alike) : TransportDelay  DelayTime=delay_a
  pos : Outport
  pos1 : Outport  Port=2
  pos2 : Outport  Port=3
  pos3 : Outport  Port=4
  pos4 : Outport  Port=5
  pos5 : Outport  Port=6
  wires:
  G(s)/3(O3) -> TD2/1
  In4/1 -> G(s)/4(In4)
  G(s)/1(O1) -> TD/1
  TD4/1 -> pos4/1
  G(s)/4(O4) -> TD3/1
  G(s)/5(O5) -> TD4/1
  TD3/1 -> pos3/1
  G(s)/6(O6) -> TD5/1
  G(s)/2(O2) -> TD1/1
  In6/1 -> G(s)/6(In6)
  In2/1 -> G(s)/2(In2)
  In1/1 -> G(s)/1(In1)
  In3/1 -> G(s)/3(In3)
  TD2/1 -> pos2/1
  TD5/1 -> pos5/1
  TD1/1 -> pos1/1
  TD/1 -> pos/1
  In5/1 -> G(s)/5(In5)

== system NewBlockFlow/Identity ==
  Input : Inport
  Input1 : Inport  Port=2
  Input2 : Inport  Port=3
  Input3 : Inport  Port=4
  Input4 : Inport  Port=5
  Input5 : Inport  Port=6
  Output : Outport
  Output1 : Outport  Port=2
  Output2 : Outport  Port=3
  Output3 : Outport  Port=4
  Output4 : Outport  Port=5
  Output5 : Outport  Port=6
  wires:
  Input/1 -> Output/1
  Input2/1 -> Output2/1
  Input4/1 -> Output4/1
  Input3/1 -> Output3/1
  Input5/1 -> Output5/1
  Input1/1 -> Output1/1

== system NewBlockFlow/PseudoDerivative ==
  Input : Inport
  Input1 : Inport  Port=2
  Input2 : Inport  Port=3
  Input3 : Inport  Port=4
  Input4 : Inport  Port=5
  Input5 : Inport  Port=6
  pseudoDer{,1..5} (6 alike) : TransferFcn  Numerator=[omegader 0]  Denominator=[1 omegader]
  Output : Outport
  Output1 : Outport  Port=2
  Output2 : Outport  Port=3
  Output3 : Outport  Port=4
  Output4 : Outport  Port=5
  Output5 : Outport  Port=6
  wires:
  Input1/1 -> pseudoDer1/1
  Input3/1 -> pseudoDer3/1
  Input5/1 -> pseudoDer5/1
  pseudoDer5/1 -> Output5/1
  pseudoDer2/1 -> Output2/1
  pseudoDer1/1 -> Output1/1
  pseudoDer/1 -> Output/1
  pseudoDer4/1 -> Output4/1
  Input2/1 -> pseudoDer2/1
  Input/1 -> pseudoDer/1
  Input4/1 -> pseudoDer4/1
  pseudoDer3/1 -> Output3/1

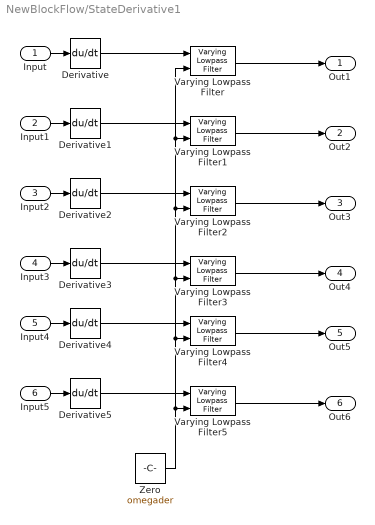
== system NewBlockFlow/StateDerivative1 ==
  Input : Inport
  Input1 : Inport  Port=2
  Input2 : Inport  Port=3
  Input3 : Inport  Port=4
  Input4 : Inport  Port=5
  Input5 : Inport  Port=6
  Derivative{,1..5} (6 alike) : Derivative
  Varying Lowpass Filter{,1..5} (6 alike) : cstblocks/Linear Parameter Varying/Varying Lowpass Filter  N=1
  Zero : Constant  Value=omegader  OutDataTypeStr=Inherit: Inherit via back propagation
  Out1 : Outport
  Out2 : Outport  Port=2
  Out3 : Outport  Port=3
  Out4 : Outport  Port=4
  Out5 : Outport  Port=5
  Out6 : Outport  Port=6
  wires:
  Input2/1 -> Derivative2/1
  Input/1 -> Derivative/1
  Input1/1 -> Derivative1/1
  Input4/1 -> Derivative4/1
  Input3/1 -> Derivative3/1
  Input5/1 -> Derivative5/1
  Derivative/1 -> Varying Lowpass Filter/1
  Derivative1/1 -> Varying Lowpass Filter1/1
  Derivative2/1 -> Varying Lowpass Filter2/1
  Derivative3/1 -> Varying Lowpass Filter3/1
  Derivative4/1 -> Varying Lowpass Filter4/1
  Derivative5/1 -> Varying Lowpass Filter5/1
  Varying Lowpass Filter/1 -> Out1/1
  Varying Lowpass Filter1/1 -> Out2/1
  Varying Lowpass Filter2/1 -> Out3/1
  Varying Lowpass Filter3/1 -> Out4/1
  Varying Lowpass Filter4/1 -> Out5/1
  Varying Lowpass Filter5/1 -> Out6/1
  Zero/1 -> Varying Lowpass Filter3/2, Varying Lowpass Filter/2, Varying Lowpass Filter1/2, Varying Lowpass Filter2/2, Varying Lowpass Filter4/2, Varying Lowpass Filter5/2

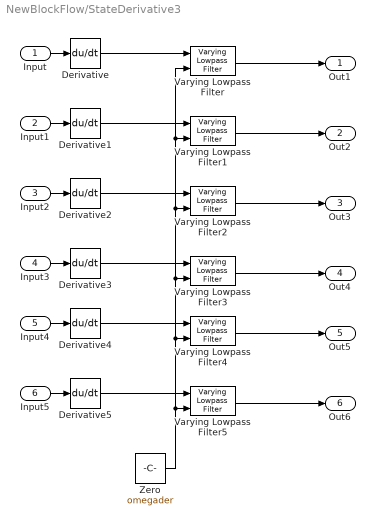
== system NewBlockFlow/StateDerivative3 ==
  Input : Inport
  Input1 : Inport  Port=2
  Input2 : Inport  Port=3
  Input3 : Inport  Port=4
  Input4 : Inport  Port=5
  Input5 : Inport  Port=6
  Derivative{,1..5} (6 alike) : Derivative
  Varying Lowpass Filter{,1..5} (6 alike) : cstblocks/Linear Parameter Varying/Varying Lowpass Filter  N=1
  Zero : Constant  Value=omegader  OutDataTypeStr=Inherit: Inherit via back propagation
  Out1 : Outport
  Out2 : Outport  Port=2
  Out3 : Outport  Port=3
  Out4 : Outport  Port=4
  Out5 : Outport  Port=5
  Out6 : Outport  Port=6
  wires:
  Input2/1 -> Derivative2/1
  Input/1 -> Derivative/1
  Input1/1 -> Derivative1/1
  Input4/1 -> Derivative4/1
  Input3/1 -> Derivative3/1
  Input5/1 -> Derivative5/1
  Derivative/1 -> Varying Lowpass Filter/1
  Derivative1/1 -> Varying Lowpass Filter1/1
  Derivative2/1 -> Varying Lowpass Filter2/1
  Derivative3/1 -> Varying Lowpass Filter3/1
  Derivative4/1 -> Varying Lowpass Filter4/1
  Derivative5/1 -> Varying Lowpass Filter5/1
  Varying Lowpass Filter/1 -> Out1/1
  Varying Lowpass Filter1/1 -> Out2/1
  Varying Lowpass Filter2/1 -> Out3/1
  Varying Lowpass Filter3/1 -> Out4/1
  Varying Lowpass Filter4/1 -> Out5/1
  Varying Lowpass Filter5/1 -> Out6/1
  Zero/1 -> Varying Lowpass Filter3/2, Varying Lowpass Filter/2, Varying Lowpass Filter1/2, Varying Lowpass Filter2/2, Varying Lowpass Filter4/2, Varying Lowpass Filter5/2

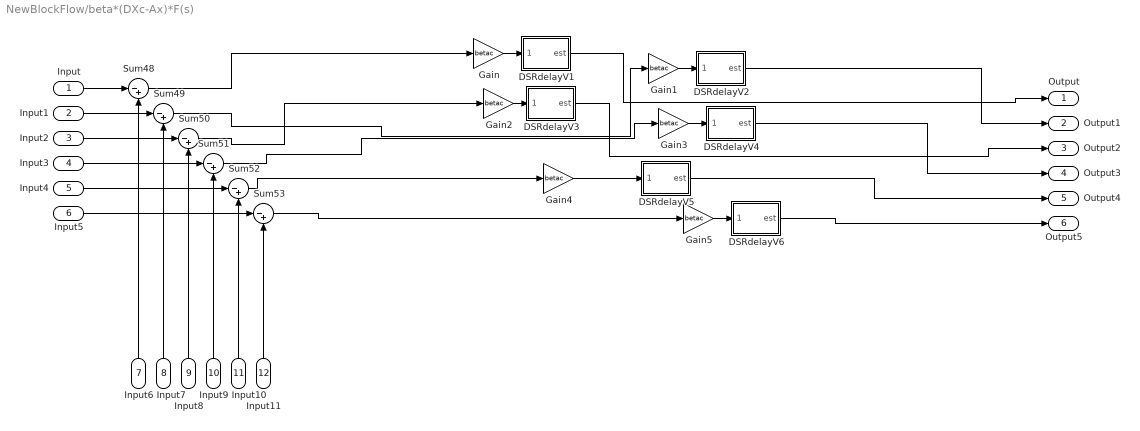
== system NewBlockFlow/beta*(DXc-Ax)*F(s) ==
  Input : Inport
  Input1 : Inport  Port=2
  Input2 : Inport  Port=3
  Input3 : Inport  Port=4
  Input4 : Inport  Port=5
  Input5 : Inport  Port=6
  Input6 : Inport  Port=7
  Input7 : Inport  Port=8
  Input8 : Inport  Port=9
  Input9 : Inport  Port=10
  Input10 : Inport  Port=11
  Input11 : Inport  Port=12
  DSRdelayV1 : Subsystem
  DSRdelayV2 : Subsystem
  DSRdelayV3 : Subsystem
  DSRdelayV4 : Subsystem
  DSRdelayV5 : Subsystem
  DSRdelayV6 : Subsystem
  Gain{,1..5} (6 alike) : Gain  Gain=betac
  Sum{48..53} (6 alike) : Sum  Inputs=|-+
  Output : Outport
  Output1 : Outport  Port=2
  Output2 : Outport  Port=3
  Output3 : Outport  Port=4
  Output4 : Outport  Port=5
  Output5 : Outport  Port=6
  wires:
  Input9/1 -> Sum51/2
  DSRdelayV2/1(est) -> Output1/1
  Gain/1 -> DSRdelayV1/1(Input)
  Gain4/1 -> DSRdelayV5/1(Input)
  Input5/1 -> Sum53/1
  Input11/1 -> Sum53/2
  Input7/1 -> Sum49/2
  Gain5/1 -> DSRdelayV6/1(Input)
  Input4/1 -> Sum52/1
  DSRdelayV5/1(est) -> Output4/1
  Sum50/1 -> Gain2/1
  Sum52/1 -> Gain4/1
  Input/1 -> Sum48/1
  Input3/1 -> Sum51/1
  Input1/1 -> Sum49/1
  Input2/1 -> Sum50/1
  DSRdelayV3/1(est) -> Output2/1
  Input6/1 -> Sum48/2
  Sum49/1 -> Gain1/1
  Sum53/1 -> Gain5/1
  Input8/1 -> Sum50/2
  Gain1/1 -> DSRdelayV2/1(Input)
  Sum51/1 -> Gain3/1
  DSRdelayV4/1(est) -> Output3/1
  Sum48/1 -> Gain/1
  Gain2/1 -> DSRdelayV3/1(Input)
  DSRdelayV6/1(est) -> Output5/1
  DSRdelayV1/1(est) -> Output/1
  Input10/1 -> Sum52/2
  Gain3/1 -> DSRdelayV4/1(Input)

== system NewBlockFlow/gain 1//a ==
  In1 : Inport
  In2 : Inport  Port=2
  In3 : Inport  Port=3
  In4 : Inport  Port=4
  In5 : Inport  Port=5
  In6 : Inport  Port=6
  1/a{,1..5} (6 alike) : Gain  Gain=1/a
  Out1 : Outport
  Out2 : Outport  Port=2
  Out3 : Outport  Port=3
  Out4 : Outport  Port=4
  Out5 : Outport  Port=5
  Out6 : Outport  Port=6
  wires:
  1/a2/1 -> Out3/1
  In1/1 -> 1/a/1
  In4/1 -> 1/a3/1
  1/a5/1 -> Out6/1
  In2/1 -> 1/a1/1
  1/a4/1 -> Out5/1
  1/a/1 -> Out1/1
  In6/1 -> 1/a5/1
  1/a3/1 -> Out4/1
  In5/1 -> 1/a4/1
  In3/1 -> 1/a2/1
  1/a1/1 -> Out2/1

== system NewBlockFlow/gain 1//a1 ==
  In1 : Inport
  In2 : Inport  Port=2
  In3 : Inport  Port=3
  In4 : Inport  Port=4
  In5 : Inport  Port=5
  In6 : Inport  Port=6
  1/a{,1..5} (6 alike) : Gain  Gain=1/a
  Out1 : Outport
  Out2 : Outport  Port=2
  Out3 : Outport  Port=3
  Out4 : Outport  Port=4
  Out5 : Outport  Port=5
  Out6 : Outport  Port=6
  wires:
  1/a2/1 -> Out3/1
  In1/1 -> 1/a/1
  In4/1 -> 1/a3/1
  1/a5/1 -> Out6/1
  In2/1 -> 1/a1/1
  1/a4/1 -> Out5/1
  1/a/1 -> Out1/1
  In6/1 -> 1/a5/1
  1/a3/1 -> Out4/1
  In5/1 -> 1/a4/1
  In3/1 -> 1/a2/1
  1/a1/1 -> Out2/1

== system NewBlockFlow/gain 1//a2 ==
  In1 : Inport
  In2 : Inport  Port=2
  In3 : Inport  Port=3
  In4 : Inport  Port=4
  In5 : Inport  Port=5
  In6 : Inport  Port=6
  1/a{,1..5} (6 alike) : Gain  Gain=1/a
  Out1 : Outport
  Out2 : Outport  Port=2
  Out3 : Outport  Port=3
  Out4 : Outport  Port=4
  Out5 : Outport  Port=5
  Out6 : Outport  Port=6
  wires:
  1/a2/1 -> Out3/1
  In1/1 -> 1/a/1
  In4/1 -> 1/a3/1
  1/a5/1 -> Out6/1
  In2/1 -> 1/a1/1
  1/a4/1 -> Out5/1
  1/a/1 -> Out1/1
  In6/1 -> 1/a5/1
  1/a3/1 -> Out4/1
  In5/1 -> 1/a4/1
  In3/1 -> 1/a2/1
  1/a1/1 -> Out2/1

== system NewBlockFlow/C(s)/C(s)1 ==
  R-F : Inport
  DSRdelayV1 : Subsystem
  Gain : Gain  Gain=betac
  Gain1 : Gain  Gain=betac*alpha^2
  Gain2 : Gain  Gain=2*alpha*betac
  Sum : Sum  Inputs=---
  pseudoDer : TransferFcn  Numerator=[omegader 0]  Denominator=[1 omegader]
  Out1 : Outport
  wires:
  Gain/1 -> DSRdelayV1/1(Input)
  Gain1/1 -> Sum/2
  Sum/1 -> Out1/1
  R-F/1 -> Gain2/1, Gain1/1, Gain/1
  DSRdelayV1/1(est) -> Sum/1
  pseudoDer/1 -> Sum/3
  Gain2/1 -> pseudoDer/1

== system NewBlockFlow/C(s)/C(s)2 ==
  R-F : Inport
  DSRdelayV1 : Subsystem
  Gain : Gain  Gain=betac
  Gain1 : Gain  Gain=betac*alpha^2
  Gain2 : Gain  Gain=2*alpha*betac
  Sum : Sum  Inputs=---
  pseudoDer : TransferFcn  Numerator=[omegader 0]  Denominator=[1 omegader]
  Out1 : Outport
  wires:
  Gain/1 -> DSRdelayV1/1(Input)
  Gain1/1 -> Sum/2
  Sum/1 -> Out1/1
  R-F/1 -> Gain2/1, Gain1/1, Gain/1
  DSRdelayV1/1(est) -> Sum/1
  pseudoDer/1 -> Sum/3
  Gain2/1 -> pseudoDer/1

== system NewBlockFlow/C(s)/C(s)3 ==
  R-F : Inport
  DSRdelayV1 : Subsystem
  Gain : Gain  Gain=betac
  Gain1 : Gain  Gain=betac*alpha^2
  Gain2 : Gain  Gain=2*alpha*betac
  Sum : Sum  Inputs=---
  pseudoDer : TransferFcn  Numerator=[omegader 0]  Denominator=[1 omegader]
  Out1 : Outport
  wires:
  Gain/1 -> DSRdelayV1/1(Input)
  Gain1/1 -> Sum/2
  Sum/1 -> Out1/1
  R-F/1 -> Gain2/1, Gain1/1, Gain/1
  DSRdelayV1/1(est) -> Sum/1
  pseudoDer/1 -> Sum/3
  Gain2/1 -> pseudoDer/1

== system NewBlockFlow/C(s)/C(s)4 ==
  R-F : Inport
  DSRdelayV1 : Subsystem
  Gain : Gain  Gain=betac
  Gain1 : Gain  Gain=betac*alpha^2
  Gain2 : Gain  Gain=2*alpha*betac
  Sum : Sum  Inputs=---
  pseudoDer : TransferFcn  Numerator=[omegader 0]  Denominator=[1 omegader]
  Out1 : Outport
  wires:
  Gain/1 -> DSRdelayV1/1(Input)
  Gain1/1 -> Sum/2
  Sum/1 -> Out1/1
  R-F/1 -> Gain2/1, Gain1/1, Gain/1
  DSRdelayV1/1(est) -> Sum/1
  pseudoDer/1 -> Sum/3
  Gain2/1 -> pseudoDer/1

== system NewBlockFlow/C(s)/C(s)5 ==
  R-F : Inport
  DSRdelayV1 : Subsystem
  Gain : Gain  Gain=betac
  Gain1 : Gain  Gain=betac*alpha^2
  Gain2 : Gain  Gain=2*alpha*betac
  Sum : Sum  Inputs=---
  pseudoDer : TransferFcn  Numerator=[omegader 0]  Denominator=[1 omegader]
  Out1 : Outport
  wires:
  Gain/1 -> DSRdelayV1/1(Input)
  Gain1/1 -> Sum/2
  Sum/1 -> Out1/1
  R-F/1 -> Gain2/1, Gain1/1, Gain/1
  DSRdelayV1/1(est) -> Sum/1
  pseudoDer/1 -> Sum/3
  Gain2/1 -> pseudoDer/1

== system NewBlockFlow/C(s)/C(s)6 ==
  R-F : Inport
  DSRdelayV1 : Subsystem
  Gain : Gain  Gain=betac
  Gain1 : Gain  Gain=betac*alpha^2
  Gain2 : Gain  Gain=2*alpha*betac
  Sum : Sum  Inputs=---
  pseudoDer : TransferFcn  Numerator=[omegader 0]  Denominator=[1 omegader]
  Out1 : Outport
  wires:
  Gain/1 -> DSRdelayV1/1(Input)
  Gain1/1 -> Sum/2
  Sum/1 -> Out1/1
  R-F/1 -> Gain2/1, Gain1/1, Gain/1
  DSRdelayV1/1(est) -> Sum/1
  pseudoDer/1 -> Sum/3
  Gain2/1 -> pseudoDer/1

== system NewBlockFlow/C(s)1/C(s)1 ==
  R-F : Inport
  Derivative : Derivative
  Gain1 : Gain  Gain=betac*alpha^2
  Gain2 : Gain  Gain=2*alpha*betac
  Sum : Sum  Inputs=|--
  Varying Lowpass Filter : cstblocks/Linear Parameter Varying/Varying Lowpass Filter  N=1
  Zero : Constant  Value=omegader  OutDataTypeStr=Inherit: Inherit via back propagation
  Out1 : Outport
  wires:
  Gain1/1 -> Sum/1
  Sum/1 -> Out1/1
  R-F/1 -> Gain2/1, Gain1/1
  Gain2/1 -> Derivative/1
  Derivative/1 -> Varying Lowpass Filter/1
  Zero/1 -> Varying Lowpass Filter/2
  Varying Lowpass Filter/1 -> Sum/2

== system NewBlockFlow/C(s)1/C(s)2 ==
  R-F : Inport
  Derivative : Derivative
  Gain1 : Gain  Gain=betac*alpha^2
  Gain2 : Gain  Gain=2*alpha*betac
  Sum : Sum  Inputs=|--
  Varying Lowpass Filter : cstblocks/Linear Parameter Varying/Varying Lowpass Filter  N=1
  Zero : Constant  Value=omegader  OutDataTypeStr=Inherit: Inherit via back propagation
  Out1 : Outport
  wires:
  Gain1/1 -> Sum/1
  Sum/1 -> Out1/1
  R-F/1 -> Gain2/1, Gain1/1
  Gain2/1 -> Derivative/1
  Derivative/1 -> Varying Lowpass Filter/1
  Zero/1 -> Varying Lowpass Filter/2
  Varying Lowpass Filter/1 -> Sum/2

== system NewBlockFlow/C(s)1/C(s)3 ==
  R-F : Inport
  Derivative : Derivative
  Gain1 : Gain  Gain=betac*alpha^2
  Gain2 : Gain  Gain=2*alpha*betac
  Sum : Sum  Inputs=|--
  Varying Lowpass Filter : cstblocks/Linear Parameter Varying/Varying Lowpass Filter  N=1
  Zero : Constant  Value=omegader  OutDataTypeStr=Inherit: Inherit via back propagation
  Out1 : Outport
  wires:
  Gain1/1 -> Sum/1
  Sum/1 -> Out1/1
  R-F/1 -> Gain2/1, Gain1/1
  Gain2/1 -> Derivative/1
  Derivative/1 -> Varying Lowpass Filter/1
  Zero/1 -> Varying Lowpass Filter/2
  Varying Lowpass Filter/1 -> Sum/2

== system NewBlockFlow/C(s)1/C(s)4 ==
  R-F : Inport
  Derivative : Derivative
  Gain1 : Gain  Gain=betac*alpha^2
  Gain2 : Gain  Gain=2*alpha*betac
  Sum : Sum  Inputs=|--
  Varying Lowpass Filter : cstblocks/Linear Parameter Varying/Varying Lowpass Filter  N=1
  Zero : Constant  Value=omegader  OutDataTypeStr=Inherit: Inherit via back propagation
  Out1 : Outport
  wires:
  Gain1/1 -> Sum/1
  Sum/1 -> Out1/1
  R-F/1 -> Gain2/1, Gain1/1
  Gain2/1 -> Derivative/1
  Derivative/1 -> Varying Lowpass Filter/1
  Zero/1 -> Varying Lowpass Filter/2
  Varying Lowpass Filter/1 -> Sum/2

== system NewBlockFlow/C(s)1/C(s)5 ==
  R-F : Inport
  Derivative : Derivative
  Gain1 : Gain  Gain=betac*alpha^2
  Gain2 : Gain  Gain=2*alpha*betac
  Sum : Sum  Inputs=|--
  Varying Lowpass Filter : cstblocks/Linear Parameter Varying/Varying Lowpass Filter  N=1
  Zero : Constant  Value=omegader  OutDataTypeStr=Inherit: Inherit via back propagation
  Out1 : Outport
  wires:
  Gain1/1 -> Sum/1
  Sum/1 -> Out1/1
  R-F/1 -> Gain2/1, Gain1/1
  Gain2/1 -> Derivative/1
  Derivative/1 -> Varying Lowpass Filter/1
  Zero/1 -> Varying Lowpass Filter/2
  Varying Lowpass Filter/1 -> Sum/2

== system NewBlockFlow/C(s)1/C(s)6 ==
  R-F : Inport
  Derivative : Derivative
  Gain1 : Gain  Gain=betac*alpha^2
  Gain2 : Gain  Gain=2*alpha*betac
  Sum : Sum  Inputs=|--
  Varying Lowpass Filter : cstblocks/Linear Parameter Varying/Varying Lowpass Filter  N=1
  Zero : Constant  Value=omegader  OutDataTypeStr=Inherit: Inherit via back propagation
  Out1 : Outport
  wires:
  Gain1/1 -> Sum/1
  Sum/1 -> Out1/1
  R-F/1 -> Gain2/1, Gain1/1
  Gain2/1 -> Derivative/1
  Derivative/1 -> Varying Lowpass Filter/1
  Zero/1 -> Varying Lowpass Filter/2
  Varying Lowpass Filter/1 -> Sum/2

== system NewBlockFlow/C(s)2/C(s)1 ==
  R-F : Inport
  DSRdelayV1 : Subsystem
  Derivative : Derivative
  Gain : Gain  Gain=betac
  Gain1 : Gain  Gain=betac*alpha^2
  Gain3 : Gain  Gain=2*alpha*betac
  Sum : Sum  Inputs=---
  Varying Lowpass Filter : cstblocks/Linear Parameter Varying/Varying Lowpass Filter  N=1
  Zero : Constant  Value=omegader  OutDataTypeStr=Inherit: Inherit via back propagation
  Out1 : Outport
  wires:
  Gain/1 -> DSRdelayV1/1(Input)
  Gain1/1 -> Sum/2
  Sum/1 -> Out1/1
  R-F/1 -> Gain3/1, Gain1/1, Gain/1
  DSRdelayV1/1(est) -> Sum/1
  Zero/1 -> Varying Lowpass Filter/2
  Varying Lowpass Filter/1 -> Sum/3
  Gain3/1 -> Derivative/1
  Derivative/1 -> Varying Lowpass Filter/1

== system NewBlockFlow/C(s)2/C(s)2 ==
  R-F : Inport
  DSRdelayV1 : Subsystem
  Derivative : Derivative
  Gain : Gain  Gain=betac
  Gain1 : Gain  Gain=betac*alpha^2
  Gain3 : Gain  Gain=2*alpha*betac
  Sum : Sum  Inputs=---
  Varying Lowpass Filter : cstblocks/Linear Parameter Varying/Varying Lowpass Filter  N=1
  Zero : Constant  Value=omegader  OutDataTypeStr=Inherit: Inherit via back propagation
  Out1 : Outport
  wires:
  Gain/1 -> DSRdelayV1/1(Input)
  Gain1/1 -> Sum/2
  Sum/1 -> Out1/1
  R-F/1 -> Gain3/1, Gain1/1, Gain/1
  DSRdelayV1/1(est) -> Sum/1
  Zero/1 -> Varying Lowpass Filter/2
  Varying Lowpass Filter/1 -> Sum/3
  Gain3/1 -> Derivative/1
  Derivative/1 -> Varying Lowpass Filter/1

== system NewBlockFlow/C(s)2/C(s)3 ==
  R-F : Inport
  DSRdelayV1 : Subsystem
  Derivative : Derivative
  Gain : Gain  Gain=betac
  Gain1 : Gain  Gain=betac*alpha^2
  Gain3 : Gain  Gain=2*alpha*betac
  Sum : Sum  Inputs=---
  Varying Lowpass Filter : cstblocks/Linear Parameter Varying/Varying Lowpass Filter  N=1
  Zero : Constant  Value=omegader  OutDataTypeStr=Inherit: Inherit via back propagation
  Out1 : Outport
  wires:
  Gain/1 -> DSRdelayV1/1(Input)
  Gain1/1 -> Sum/2
  Sum/1 -> Out1/1
  R-F/1 -> Gain3/1, Gain1/1, Gain/1
  DSRdelayV1/1(est) -> Sum/1
  Zero/1 -> Varying Lowpass Filter/2
  Varying Lowpass Filter/1 -> Sum/3
  Gain3/1 -> Derivative/1
  Derivative/1 -> Varying Lowpass Filter/1

== system NewBlockFlow/C(s)2/C(s)4 ==
  R-F : Inport
  DSRdelayV1 : Subsystem
  Derivative : Derivative
  Gain : Gain  Gain=betac
  Gain1 : Gain  Gain=betac*alpha^2
  Gain3 : Gain  Gain=2*alpha*betac
  Sum : Sum  Inputs=---
  Varying Lowpass Filter : cstblocks/Linear Parameter Varying/Varying Lowpass Filter  N=1
  Zero : Constant  Value=omegader  OutDataTypeStr=Inherit: Inherit via back propagation
  Out1 : Outport
  wires:
  Gain/1 -> DSRdelayV1/1(Input)
  Gain1/1 -> Sum/2
  Sum/1 -> Out1/1
  R-F/1 -> Gain3/1, Gain1/1, Gain/1
  DSRdelayV1/1(est) -> Sum/1
  Zero/1 -> Varying Lowpass Filter/2
  Varying Lowpass Filter/1 -> Sum/3
  Gain3/1 -> Derivative/1
  Derivative/1 -> Varying Lowpass Filter/1

== system NewBlockFlow/C(s)2/C(s)5 ==
  R-F : Inport
  DSRdelayV1 : Subsystem
  Derivative : Derivative
  Gain : Gain  Gain=betac
  Gain1 : Gain  Gain=betac*alpha^2
  Gain3 : Gain  Gain=2*alpha*betac
  Sum : Sum  Inputs=---
  Varying Lowpass Filter : cstblocks/Linear Parameter Varying/Varying Lowpass Filter  N=1
  Zero : Constant  Value=omegader  OutDataTypeStr=Inherit: Inherit via back propagation
  Out1 : Outport
  wires:
  Gain/1 -> DSRdelayV1/1(Input)
  Gain1/1 -> Sum/2
  Sum/1 -> Out1/1
  R-F/1 -> Gain3/1, Gain1/1, Gain/1
  DSRdelayV1/1(est) -> Sum/1
  Zero/1 -> Varying Lowpass Filter/2
  Varying Lowpass Filter/1 -> Sum/3
  Gain3/1 -> Derivative/1
  Derivative/1 -> Varying Lowpass Filter/1

== system NewBlockFlow/C(s)2/C(s)6 ==
  R-F : Inport
  DSRdelayV1 : Subsystem
  Derivative : Derivative
  Gain : Gain  Gain=betac
  Gain1 : Gain  Gain=betac*alpha^2
  Gain3 : Gain  Gain=2*alpha*betac
  Sum : Sum  Inputs=---
  Varying Lowpass Filter : cstblocks/Linear Parameter Varying/Varying Lowpass Filter  N=1
  Zero : Constant  Value=omegader  OutDataTypeStr=Inherit: Inherit via back propagation
  Out1 : Outport
  wires:
  Gain/1 -> DSRdelayV1/1(Input)
  Gain1/1 -> Sum/2
  Sum/1 -> Out1/1
  R-F/1 -> Gain3/1, Gain1/1, Gain/1
  DSRdelayV1/1(est) -> Sum/1
  Zero/1 -> Varying Lowpass Filter/2
  Varying Lowpass Filter/1 -> Sum/3
  Gain3/1 -> Derivative/1
  Derivative/1 -> Varying Lowpass Filter/1
